simulink model "planta_sensores_CA"  (R2025b)
settings: Solver=VariableStepAuto  StartTime=0.0  StopTime=10  RelTol=1e-2
model workspace (MAT data in the model file):
  w = 0.5
values from neighbouring files (symbols this model uses):
  C1 = 1.2801    [Data_ControleLateral_atual.m]
  C2 = 23.99    [Data_ControleLateral_atual.m]
  C3 = 0.52    [Data_ControleLateral_atual.m]
undefined symbols (not defined in the file or in its folder): EV, GND, MTR
libraries: autolibshared x5, autolibutils x4, sharedtransform x4, simulink x3, autolibmappedmotor x2, vehdynlibviscommon x1, slpidlib x1, vehdynlibdriver x1, vehdynlibsens x1
(part 3 of 3)

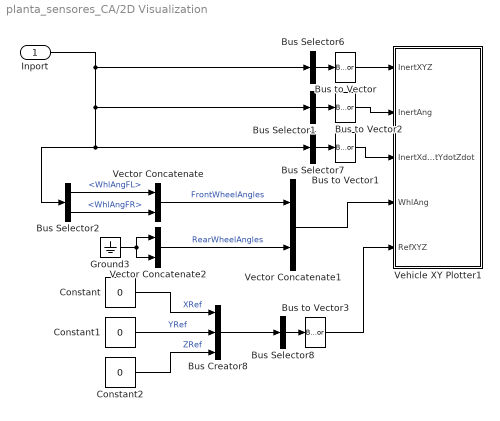
== system planta_sensores_CA/2D Visualization ==
  Inport : Inport
  Bus Creator8 : BusCreator  Inputs=3
  Bus Selector1 : BusSelector  OutputSignals=InertFrm.Cg.Ang.phi,InertFrm.Cg.Ang.theta,InertFrm.Cg.Ang.psi  OutputAsBus=on
  Bus Selector2 : BusSelector  OutputSignals=BdyFrm.FrntAxl.Steer.WhlAngFL,BdyFrm.FrntAxl.Steer.WhlAngFR
  Bus Selector6 : BusSelector  OutputSignals=InertFrm.Geom.Disp.X,InertFrm.Geom.Disp.Y,InertFrm.Geom.Disp.Z  OutputAsBus=on
  Bus Selector7 : BusSelector  OutputSignals=InertFrm.Geom.Vel.Xdot,InertFrm.Geom.Vel.Ydot,InertFrm.Geom.Vel.Zdot  OutputAsBus=on
  Bus Selector8 : BusSelector  OutputSignals=XRef,YRef,ZRef  OutputAsBus=on
  Bus to Vector{,1..3} (4 alike) : BusToVector
  Constant : Constant  Value=0
  Constant1 : Constant  Value=0
  Constant2 : Constant  Value=0
  Ground3 : Ground
  Vector Concatenate : Concatenate
  Vector Concatenate1 : Concatenate
  Vector Concatenate2 : Concatenate
  Vehicle XY Plotter1 : Subsystem  mask(Vehicle XY Plotter){extRef=on, extStats=off, extTireF=off, a=EV.FrontAxlePositionfromCG, b=EV.RearAxlePositionfromCG, w=1.17, figBorder=10, bufferSize=1024, velNorm=5, tireFNorm=1000, pltDT=0.1}
      mask prompts: extRef "Plot path reference, extRef"; extStats "Display speed, RPM and Gear"; extTireF "Display tire forces"; a "Distance to front axle from CG, a [m]:"; b "Distance to rear axle from CG, b [m]:"; w "Track width, w [m]:"; figBorder "Distance to figure borders, figBorder [m]:"; bufferSize "Path buffer sampe size, bufferSize []:"; velNorm "Velocity vector scaling, velNorm [m*s/m]:"; tireFNorm "Tire force vector scaling, tireFNorm [m/N]:"; pltDT "Plot update rate, pltDT [s]:"
      mask help:
      | This block will display a MATLAB figure which indicates the vehicle path, current position and heading velocity.
      | An optional path reference is also provided.
      mask init:
      | block = gcb;
      | if autoblkschecksimstopped(block)
      |     ParamNames = {'extRef';'extStats';'extTireF';'extTireF'};
      |     PortNames = {'RefXYZ';'Stats';'TireFx';'TireFy'};
      |     for idx=1:length(PortNames)
      |         InportOption  = {'built-in/Ground', [PortNames{idx}, ' Ground'];...
      |             'built-in/Inport',PortNames{idx}};
      |         if ~strcmp(get_param(block,ParamNames{idx}),'on')
      |             NewBlkHdl = autoblksreplaceblock(block, InportOption, 1);
      |             set_param(NewBlkHdl, 'ShowName', 'off');
      |         else
      |             autoblksreplaceblock(block, InportOption, 2);
      |         end
      |     end
      |     InportNames = {'InertXYZ';'InertAng';'InertXdotYdotZdot';'WhlAng';'RefXYZ';'Stats';'TireFx';'TireFy'};
      |     FoundNames = get_param(find_system(block, 'LookUnderMasks', 'all', 'SearchDepth', 1, 'FollowLinks', 'on', 'BlockType', 'Inport'), 'Name');
      |     [~,PortI] = intersect(InportNames, FoundNames);
      |     PortI = sort(PortI);
      |     for idx = 1:length(PortI)
      |         set_param([block, '/', InportNames{PortI(idx)}], 'Port', num2str(idx));
      |     end
      | end
      mask TypeOptions a: Vehicle XY Plotter/a
      mask TypeOptions b: Vehicle XY Plotter/b
      mask TypeOptions w: Vehicle XY Plotter/w
      mask TypeOptions figBorder: Vehicle XY Plotter/figBorder
      mask TypeOptions bufferSize: Vehicle XY Plotter/bufferSize
      mask TypeOptions velNorm: Vehicle XY Plotter/velNorm
      mask TypeOptions tireFNorm: Vehicle XY Plotter/tireFNorm
      mask DialogControl Container3 Prompt: Plot and Display Options
  wires:
  Vector Concatenate1/1 -> Vehicle XY Plotter1/4(WhlAng)
  Ground3/1 -> Vector Concatenate2/1, Vector Concatenate2/2
  Bus Selector6/1 -> Bus to Vector/1
  Vector Concatenate/1 -> Vector Concatenate1/1  "FrontWheelAngles"
  Vector Concatenate2/1 -> Vector Concatenate1/2  "RearWheelAngles"
  Bus Selector7/1 -> Bus to Vector1/1
  Bus to Vector1/1 -> Vehicle XY Plotter1/3(InertXdotYdotZdot)
  Bus to Vector/1 -> Vehicle XY Plotter1/1(InertXYZ)
  Bus to Vector2/1 -> Vehicle XY Plotter1/2(InertAng)
  Bus Selector1/1 -> Bus to Vector2/1
  Inport/1 -> Bus Selector7/1, Bus Selector2/1, Bus Selector1/1, Bus Selector6/1
  Bus Selector2/1 -> Vector Concatenate/1  "<WhlAngFL>"
  Bus Selector2/2 -> Vector Concatenate/2  "<WhlAngFR>"
  Bus Creator8/1 -> Bus Selector8/1
  Bus Selector8/1 -> Bus to Vector3/1
  Constant2/1 -> Bus Creator8/3  "ZRef"
  Constant1/1 -> Bus Creator8/2  "YRef"
  Bus to Vector3/1 -> Vehicle XY Plotter1/5(RefXYZ)
  Constant/1 -> Bus Creator8/1  "XRef"

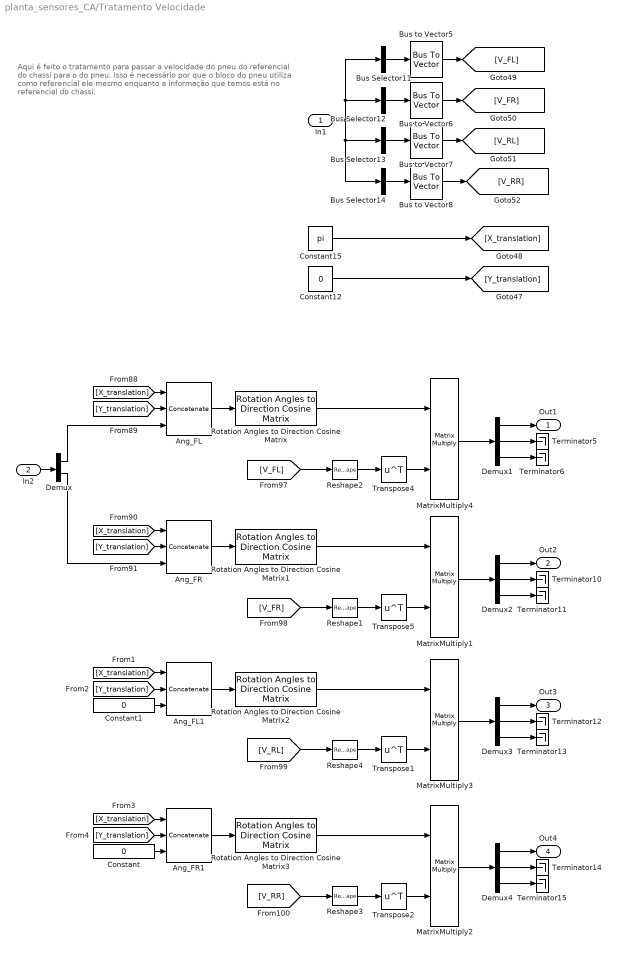
== system planta_sensores_CA/Tratamento Velocidade ==
  note: Aqui é feito o tratamento para passar a velocidade do pneu do referencial do chassi para o do pneu. Isso é necessário por que o bloco do pneu utiliza como referencial ele mesmo enquanto a informação que temos está no referencial do chassi.
  In1 : Inport
  In2 : Inport  Port=2
  Ang_FL : Concatenate  NumInputs=3  ConcatenateDimension=2
  Ang_FL1 : Concatenate  NumInputs=3  ConcatenateDimension=2
  Ang_FR : Concatenate  NumInputs=3  ConcatenateDimension=2
  Ang_FR1 : Concatenate  NumInputs=3  ConcatenateDimension=2
  Bus Selector11 : BusSelector  OutputSignals=BdyFrm.FrntAxl.Lft.Vel.xdot,BdyFrm.FrntAxl.Lft.Vel.ydot,BdyFrm.FrntAxl.Lft.Vel.zdot  OutputAsBus=on
  Bus Selector12 : BusSelector  OutputSignals=BdyFrm.FrntAxl.Rght.Vel.xdot,BdyFrm.FrntAxl.Rght.Vel.ydot,BdyFrm.FrntAxl.Rght.Vel.zdot  OutputAsBus=on
  Bus Selector13 : BusSelector  OutputSignals=BdyFrm.RearAxl.Lft.Vel.xdot,BdyFrm.RearAxl.Lft.Vel.ydot,BdyFrm.RearAxl.Lft.Vel.zdot  OutputAsBus=on
  Bus Selector14 : BusSelector  OutputSignals=BdyFrm.RearAxl.Rght.Vel.xdot,BdyFrm.RearAxl.Rght.Vel.ydot,BdyFrm.RearAxl.Rght.Vel.zdot  OutputAsBus=on
  Bus to Vector{5..8} (4 alike) : BusToVector
  Constant : Constant  Value=0
  Constant1 : Constant  Value=0
  Constant12 : Constant  Value=0
  Constant15 : Constant  Value=pi
  Demux : Demux  Outputs=2
  Demux{1..4} (4 alike) : Demux  Outputs=3
  MatrixMultiply{1..4} (4 alike) : Product  Multiplication=Matrix(*)
  Reshape{1..4} (4 alike) : Reshape  OutputDimensionality=Row vector (2-D)
  Rotation Angles to Direction Cosine Matrix{,1..3} (4 alike) : sharedtransform/Rotation Angles to Direction Cosine Matrix  rotationOrder=XYZ  aMode=2
  Terminator{5..6,10..15} (8 alike) : Terminator
  Transpose{1..2,4..5} (4 alike) : Math  Operator=transpose
  Out1 : Outport
  Out2 : Outport  Port=2
  Out3 : Outport  Port=3
  Out4 : Outport  Port=4
  wires:
  Demux1/3 -> Terminator6/1
  Demux3/3 -> Terminator13/1
  Ang_FL/1 -> Rotation Angles to Direction Cosine Matrix/1
  Demux4/3 -> Terminator15/1
  Bus to Vector6/1 -> [V_FR]
  Transpose4/1 -> MatrixMultiply4/2
  Demux4/2 -> Terminator14/1
  Constant15/1 -> [X_translation]
  Bus to Vector7/1 -> [V_RL]
  In2/1 -> Demux/1
  Rotation Angles to Direction Cosine Matrix/1 -> MatrixMultiply4/1
  [V_FL] -> Reshape2/1
  MatrixMultiply1/1 -> Demux2/1
  Demux3/2 -> Terminator12/1
  Demux2/3 -> Terminator11/1
  Reshape1/1 -> Transpose5/1
  Demux/1 -> Ang_FL/3
  In1/1 -> Bus Selector13/1, Bus Selector14/1, Bus Selector12/1, Bus Selector11/1
  Ang_FR/1 -> Rotation Angles to Direction Cosine Matrix1/1
  Constant12/1 -> [Y_translation]
  Reshape2/1 -> Transpose4/1
  Bus to Vector5/1 -> [V_FL]
  [X_translation] -> Ang_FL/1
  [X_translation] -> Ang_FR/1
  Demux/2 -> Ang_FR/3
  Bus Selector12/1 -> Bus to Vector6/1
  Bus Selector13/1 -> Bus to Vector7/1
  Bus Selector14/1 -> Bus to Vector8/1
  [V_FR] -> Reshape1/1
  Transpose5/1 -> MatrixMultiply1/2
  Bus to Vector8/1 -> [V_RR]
  [Y_translation] -> Ang_FR/2
  [Y_translation] -> Ang_FL/2
  MatrixMultiply4/1 -> Demux1/1
  Demux2/2 -> Terminator10/1
  Demux3/1 -> Out3/1
  Demux1/2 -> Terminator5/1
  Demux2/1 -> Out2/1
  Demux4/1 -> Out4/1
  Bus Selector11/1 -> Bus to Vector5/1
  Rotation Angles to Direction Cosine Matrix1/1 -> MatrixMultiply1/1
  Demux1/1 -> Out1/1
  Rotation Angles to Direction Cosine Matrix3/1 -> MatrixMultiply2/1
  Reshape4/1 -> Transpose1/1
  [Y_translation] -> Ang_FL1/2
  Transpose2/1 -> MatrixMultiply2/2
  Reshape3/1 -> Transpose2/1
  [Y_translation] -> Ang_FR1/2
  Rotation Angles to Direction Cosine Matrix2/1 -> MatrixMultiply3/1
  MatrixMultiply2/1 -> Demux4/1
  Transpose1/1 -> MatrixMultiply3/2
  [X_translation] -> Ang_FL1/1
  MatrixMultiply3/1 -> Demux3/1
  Ang_FL1/1 -> Rotation Angles to Direction Cosine Matrix2/1
  Ang_FR1/1 -> Rotation Angles to Direction Cosine Matrix3/1
  [X_translation] -> Ang_FR1/1
  [V_RR] -> Reshape3/1
  [V_RL] -> Reshape4/1
  Constant/1 -> Ang_FR1/3
  Constant1/1 -> Ang_FL1/3

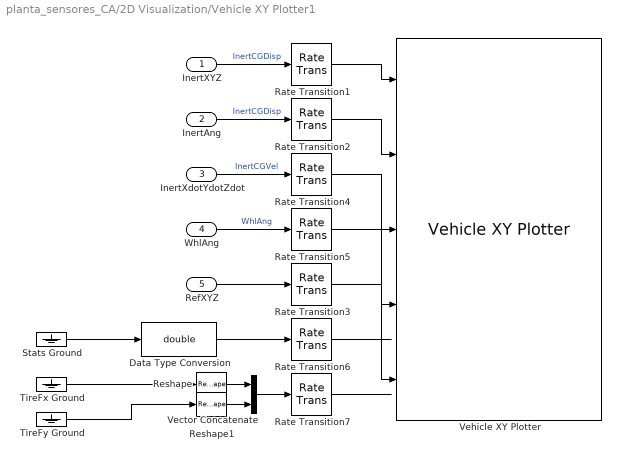
== system planta_sensores_CA/2D Visualization/Vehicle XY Plotter1 ==
  InertXYZ : Inport
  InertAng : Inport  Port=2
  InertXdotYdotZdot : Inport  Port=3
  WhlAng : Inport  Port=4
  RefXYZ : Inport  Port=5
  Data Type Conversion : DataTypeConversion  OutDataTypeStr=double  SaturateOnIntegerOverflow=off  RndMeth=Floor
  Rate Transition{1..7} (7 alike) : RateTransition  Deterministic=off  OutPortSampleTime=pltDT
  Reshape : Reshape  OutputDimensionality=Row vector (2-D)
  Reshape1 : Reshape  OutputDimensionality=Row vector (2-D)
  Stats Ground : Ground
  TireFx Ground : Ground
  TireFy Ground : Ground
  Vector Concatenate : Concatenate  Mode=Multidimensional array
  Vehicle XY Plotter : vehdynlibviscommon/Vehicle XY Plotter  w=w  a=a  b=b  figBorder=figBorder  bufferSize=bufferSize  extStats=off  extTireF=off
  wires:
  Vector Concatenate/1 -> Rate Transition7/1
  Reshape1/1 -> Vector Concatenate/2
  Reshape/1 -> Vector Concatenate/1
  RefXYZ/1 -> Rate Transition3/1
  Rate Transition7/1 -> ?
  Data Type Conversion/1 -> Rate Transition6/1
  Rate Transition6/1 -> ?
  Rate Transition5/1 -> Vehicle XY Plotter/4
  Rate Transition4/1 -> Vehicle XY Plotter/3
  Rate Transition2/1 -> Vehicle XY Plotter/2
  Rate Transition1/1 -> Vehicle XY Plotter/1
  Rate Transition3/1 -> Vehicle XY Plotter/5
  WhlAng/1 -> Rate Transition5/1  "WhlAng"
  InertXYZ/1 -> Rate Transition1/1  "InertCGDisp"
  InertXdotYdotZdot/1 -> Rate Transition4/1  "InertCGVel"
  InertAng/1 -> Rate Transition2/1  "InertCGDisp"
  Stats Ground/1 -> Data Type Conversion/1
  TireFx Ground/1 -> Reshape/1
  TireFy Ground/1 -> Reshape1/1

== matlab function planta_sensores_CA/MATLAB Function1 ==
  data: Vcg input; SR_L output; RL_speed input; RR_speed input; SR_R output
function [SR_L, SR_R] = fcn(Vcg, RL_speed, RR_speed)
%#codegen

% --- Configuração de Segurança ---
% 'epsilon' é um valor pequeno que impede a divisão por zero.
% 0.1 m/s é um bom valor: abaixo disso, consideramos "parado".
epsilon = 0.1; 

% --- Slip Esquerdo (SR_L) ---
% A fórmula é: (V_roda - V_carro) / V_roda
% Truque: O denominador será o MAIOR valor entre 'a velocidade real' e '0.1'.
% Se a roda estiver parada (0), ele usa 0.1. Se estiver a 10, usa 10.
denominador_L = max(abs(Vcg), epsilon);

SR_L = ((RL_speed*0.25) - Vcg) / denominador_L;


% --- Slip Direito (SR_R) ---
denominador_R = max(abs(Vcg), epsilon);

SR_R = ((RR_speed*0.25) - Vcg) / denominador_R;

end

== matlab function planta_sensores_CA/MATLAB Function ==
  data: u input; vec output
function vec= fcn(u)

vec = [u(1), u(2); u(3), u(4)];

== matlab function planta_sensores_CA/MATLAB Function2 ==
  data: SR_L input; Atrito_L output; C1 input; C2 input; C3 input
function Atrito_L = fcn(SR_L, C1, C2, C3)

Atrito_L = (C1*(1-(exp(SR_L*C2*(-1)))))-(C3*SR_L);

== matlab function planta_sensores_CA/MATLAB Function3 ==
  data: SR_R input; Atrito_R output; C1 input; C2 input; C3 input
function Atrito_R = fcn(SR_R, C1, C2, C3)

Atrito_R = (C1*(1-(exp(SR_R*C2*(-1)))))-(C3*SR_R);

== matlab function planta_sensores_CA/MATLAB Function4 ==
  settings: updateMethod=DISCRETE
  data: distancia input; tempo_final output; tempo_atual input; signal output
function [tempo_final, signal]= fcn(distancia, tempo_atual)

signal = 0;
persistent tempo_registrado cruzou_linha

if isempty(tempo_registrado)
    tempo_registrado = 0;
    cruzou_linha = false;
end

if distancia >= 75 && cruzou_linha == false
    tempo_registrado = tempo_atual; 
    cruzou_linha = true;           
end

if cruzou_linha

    tempo_final = tempo_registrado; 
    signal = 1;
else
    tempo_final = 0; 
end

end

== matlab function planta_sensores_CA/MATLAB Function6 ==
  data: left_wheel_angle output; steering_angle input; right_wheel_angle output
function [left_wheel_angle, right_wheel_angle] = fcn(steering_angle)

if(steering_angle<=0)
    left_wheel_angle = 0.30732918494924799*steering_angle;
    right_wheel_angle = 0.268948751217872*steering_angle;

else (steering_angle>0)
    left_wheel_angle = 0.268948678266664*steering_angle;
    right_wheel_angle = 0.30732915888671*steering_angle;
end
end

== matlab function planta_sensores_CA/MATLAB Function7 ==
  data: setpoint input; SR_L input; SR_R input; CA_error output
function CA_error= fcn(setpoint,SR_L, SR_R)

    CA_error_left = setpoint-SR_L;

    CA_error_right = setpoint-SR_R;

    CA_error = (CA_error_left + CA_error_right)/2;

end

== matlab function planta_sensores_CA/MATLAB Function9 ==
  data: s input; x_ref output; T input; y_ref output; psi_ref output
function [x_ref, y_ref, psi_ref] = fcn(s, T)

if s <= T
    x_ref = T;

else
    x_ref = T + s;

end

y_ref = 0;
psi_ref = 0;

end
